simulink model "lab_5_task_1_simulink"  (R2025b)
settings: Solver=ode5  StartTime=0.0  StopTime=10.0  FixedStep=0.1  RelTol=1e-3
values from neighbouring files (symbols this model uses):
  A0 = eye(3)    [lab_4_task_1.m]    (also in lab_5_task_1.m; lab_5_task_2.m)
  I = diag([ix iy iz])    [lab_4_task_1.m]    (also in lab_5_task_1.m; lab_5_task_2.m; lab_6_task_1.m = diag([ ix iy iz ]); lab_6_task_2.m = diag([ ix iy iz ]))
  phi0 = 0.1    [lab_5_task_1.m]    (also in lab_5_task_2.m = 0)
  psi0 = 0.2    [lab_5_task_1.m]    (also in lab_5_task_2.m = 0)
  theta0 = 0.3    [lab_5_task_1.m]    (also in lab_5_task_2.m = 0)
  w0 = [0.01 0.01 0.01]    [lab_3_task_3.m]    (also in lab_5_task_1.m = [wx0 wy0 wz0]; lab_5_task_2.m = [wx0 wy0 wz0]; lab_6_task_1.m = [wx0 wy0 wz0]; lab_6_task_2.m = [wx0 wy0 wz0])
libraries: matrix_library x1
settings Model: Creator=nicol  LastModifiedBy=nicol

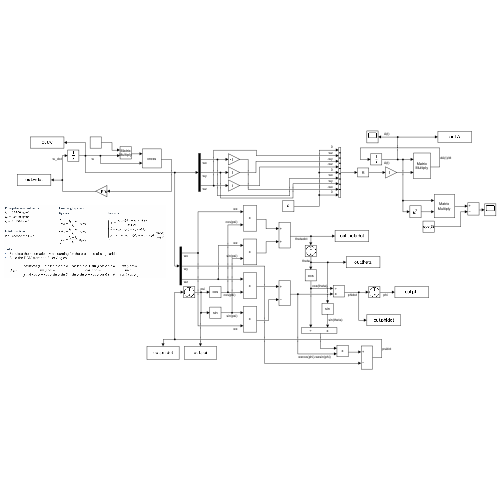
[thumbnail: Simulink's stored preview of the top-level diagram]
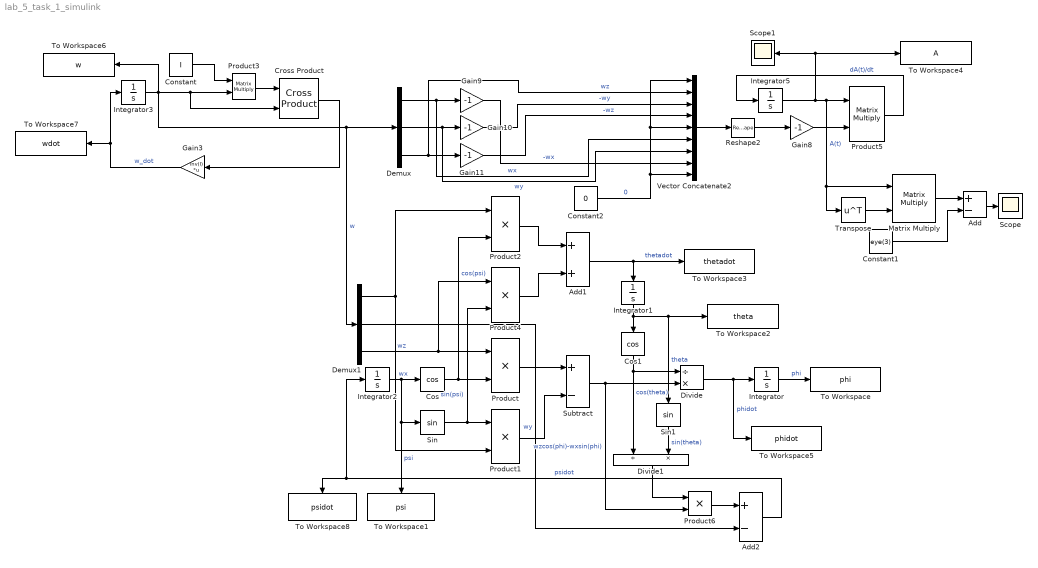
== system lab_5_task_1_simulink ==
  Add : Sum  Inputs=+-
  Add1 : Sum
  Add2 : Sum  Inputs=+-
  Constant : Constant  Value=I
  Constant1 : Constant  Value=eye(3)
  Constant2 : Constant  Value=0
  Cos : Trigonometry  Operator=cos
  Cos1 : Trigonometry  Operator=cos
  Cross Product : matrix_library/Cross Product
  Demux : Demux  Outputs=3
  Demux1 : Demux  Outputs=3
  Divide : Product  Inputs=/*
  Divide1 : Product  Inputs=/*
  Gain{8..11} (4 alike) : Gain  Gain=-1
  Gain3 : Gain  Gain=inv(I)  Multiplication=Matrix(K*u)
  Integrator : Integrator  InitialCondition=phi0  WrapState=on
  Integrator1 : Integrator  InitialCondition=theta0  WrapState=on
  Integrator2 : Integrator  InitialCondition=psi0  WrapState=on
  Integrator3 : Integrator  InitialCondition=w0
  Integrator5 : Integrator  InitialCondition=A0
  Matrix Multiply : Product  Multiplication=Matrix(*)
  Product{,1..2,4,6} (5 alike) : Product
  Product3 : Product  Multiplication=Matrix(*)
  Product5 : Product  Multiplication=Matrix(*)
  Reshape2 : Reshape  OutputDimensionality=Customize  OutputDimensions=[3,3]
  Scope : Scope
      settings: ActiveDisplayYMinimum=-6.807770444899007E-8  ActiveDisplayYMaximum=8.9871029145736092E-8
  Scope1 : Scope
      settings: ActiveDisplayYMinimum=-1  ActiveDisplayYMaximum=1
  Sin : Trigonometry
  Sin1 : Trigonometry
  Subtract : Sum  Inputs=+-
  To Workspace : ToWorkspace  VariableName=phi  SaveFormat=Timeseries  SampleTime=-1
  To Workspace1 : ToWorkspace  VariableName=psi  SaveFormat=Timeseries  SampleTime=-1
  To Workspace2 : ToWorkspace  VariableName=theta  SaveFormat=Timeseries  SampleTime=-1
  To Workspace3 : ToWorkspace  VariableName=thetadot  SaveFormat=Timeseries  SampleTime=-1
  To Workspace4 : ToWorkspace  VariableName=A  SaveFormat=Timeseries  SampleTime=-1
  To Workspace5 : ToWorkspace  VariableName=phidot  SaveFormat=Timeseries  SampleTime=-1
  To Workspace6 : ToWorkspace  VariableName=w  SaveFormat=Timeseries  SampleTime=-1
  To Workspace7 : ToWorkspace  VariableName=wdot  SaveFormat=Timeseries  SampleTime=-1
  To Workspace8 : ToWorkspace  VariableName=psidot  SaveFormat=Timeseries  SampleTime=-1
  Transpose : Math  Operator=transpose
  Vector Concatenate2 : Concatenate  NumInputs=9
  wires:
  Product5/1 -> Integrator5/1  "dA(t)/dt"
  Matrix Multiply/1 -> Add/1
  Demux/1 -> Vector Concatenate2/6, Gain9/1  "wx"
  Constant1/1 -> Add/2
  Gain3/1 -> Integrator3/1, To Workspace7/1  "w_dot"
  Add/1 -> Scope/1
  Product3/1 -> Cross Product/1
  Cross Product/1 -> Gain3/1
  Gain8/1 -> Product5/2
  Constant2/1 -> Vector Concatenate2/1, Vector Concatenate2/5, Vector Concatenate2/9  "0"
  Constant/1 -> Product3/1
  Integrator3/1 -> Demux/1, Demux1/1, Cross Product/2, Product3/2, To Workspace6/1  "w"
  Demux/2 -> Vector Concatenate2/7, Gain10/1  "wy"
  Gain10/1 -> Vector Concatenate2/3  "-wy"
  Transpose/1 -> Matrix Multiply/2
  Vector Concatenate2/1 -> Reshape2/1
  Integrator5/1 -> To Workspace4/1, Scope1/1, Transpose/1, Matrix Multiply/1, Product5/1  "A(t)"
  Demux/3 -> Vector Concatenate2/2, Gain11/1  "wz"
  Gain9/1 -> Vector Concatenate2/8  "-wx"
  Reshape2/1 -> Gain8/1
  Gain11/1 -> Vector Concatenate2/4  "-wz"
  Demux1/2 -> Add2/2  "wy"
  Demux1/3 -> Product4/1, Product/1  "wz"
  Integrator2/1 -> Sin/1, To Workspace1/1, Cos/1  "psi"
  Cos/1 -> Product/2, Product2/2  "cos(psi)"
  Product/1 -> Subtract/1
  Subtract/1 -> Product6/2, Divide/2  "wzcos(phi)-wxsin(phi)"
  Sin/1 -> Product4/2, Product1/1  "sin(psi)"
  Demux1/1 -> Product2/1, Product1/2  "wx"
  Product1/1 -> Subtract/2
  Divide/1 -> Integrator/1, To Workspace5/1  "phidot"
  Integrator/1 -> To Workspace/1  "phi"
  Product2/1 -> Add1/1
  Product4/1 -> Add1/2
  Add1/1 -> To Workspace3/1, Integrator1/1  "thetadot"
  Integrator1/1 -> To Workspace2/1, Sin1/1, Cos1/1  "theta"
  Cos1/1 -> Divide/1, Divide1/1  "cos(theta)"
  Sin1/1 -> Divide1/2  "sin(theta)"
  Product6/1 -> Add2/1
  Divide1/1 -> Product6/1
  Add2/1 -> To Workspace8/1, Integrator2/1  "psidot"
